simulink model "dwa_obstacle_avoidance"  (R2023b)
settings: Solver=VariableStepAuto  StartTime=0.0  StopTime=30  RelTol=1e-3
InitFcn:
  | if (isempty(target))
  | %load map
  | load exampleMaps simpleMap
  | mapMatrix = img_logical;
  | mapScale = 1;
  | 
  | % Max speed parameters
  | maxLinSpeed = 1.5;
  | maxAngle = deg2rad(45);
  | maxAngSpeed = 0.3;
  | 
  | % Initial pose of the robot
  | initX = 7;
  | initY = 22;
  | initTheta = pi;
  | v0=0;
  | w0=0;
  | 
  | % range sensor parameters
  | scanAngles = -pi/2:pi/128:pi/2;
  | maxRange = 12;
  | lidarNoiseVariance = 0.1^2;
  | lidarNoiseSeeds = randi(intmax,size(scanAngles));
  | 
  | %simulation parameters
  | sampleTime=0.05;
  | target = [25;5];
  | wheelBase=1.4;
  | end
values from neighbouring files (symbols this model uses):
  k1 = 0.80    (= 0.8)    [dynamic_window_init.m]    (also in sequence_dynamic_window_init.m = 0.9)
  k2 = 0.006    [dynamic_window_init.m]    (also in sequence_dynamic_window_init.m)
  k3 = 0.02    [dynamic_window_init.m]    (also in sequence_dynamic_window_init.m = 0.1)
libraries: robotmobilelib x1
settings Model: Creator=lucia  LastModifiedBy=lucia

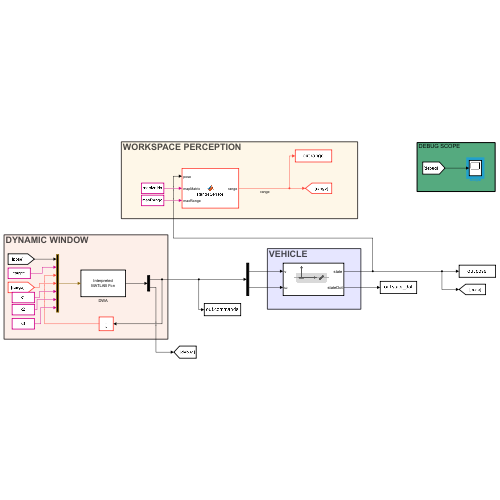
[thumbnail: Simulink's stored preview of the top-level diagram]
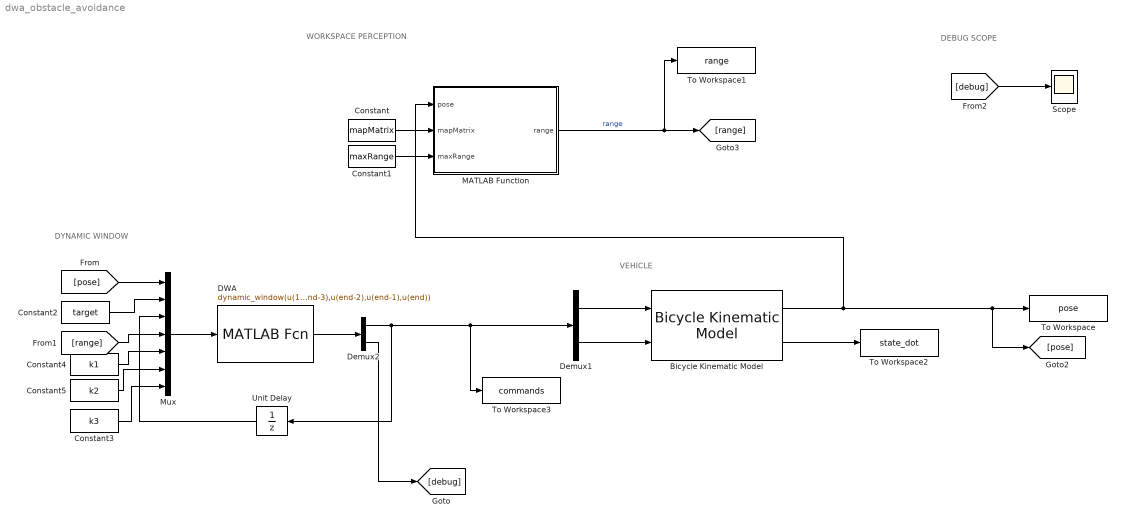
== system dwa_obstacle_avoidance ==
  note: DEBUG SCOPE
  note: DYNAMIC WINDOW
  note: VEHICLE
  note: WORKSPACE PERCEPTION
  Bicycle Kinematic Model : robotmobilelib/Bicycle Kinematic Model  VehicleInputs=Vehicle Speed & Heading Angular Velocity  WheelBase=wheelBase  VehicleSpeedRange=[0 maxLinSpeed]  MaxSteeringAngle=maxAngle  InitialState=[initX, initY, initTheta]  SimulateUsing=Interpreted execution
  Constant : Constant  Value=mapMatrix
  Constant1 : Constant  Value=maxRange
  Constant2 : Constant  Value=target
  Constant3 : Constant  Value=k3
  Constant4 : Constant  Value=k1
  Constant5 : Constant  Value=k2
  DWA : MATLABFcn  MATLABFcn=dynamic_window(u(1:3),u(4:5),u(6:7),u(8:end-3),u(end-2),u(end-1),u(end))  OutputDimensions=5
  Demux1 : Demux  Outputs=2
  Demux2 : Demux  Outputs=[2 3]
  MATLAB Function : MATLAB Function  TreatAsAtomicUnit=on
  Mux : Mux  Inputs=7
  Scope : Scope
  To Workspace : ToWorkspace  VariableName=pose  SampleTime=-1
      settings: Save2DSignal=2-D array (concatenate along first dimension)
  To Workspace1 : ToWorkspace  VariableName=range  SampleTime=-1
  To Workspace2 : ToWorkspace  VariableName=state_dot  SampleTime=-1
      settings: Save2DSignal=2-D array (concatenate along first dimension)
  To Workspace3 : ToWorkspace  VariableName=commands  SampleTime=-1
      settings: Save2DSignal=2-D array (concatenate along first dimension)
  Unit Delay : UnitDelay  InitialCondition=[v0; w0]  SampleTime=sampleTime  HasFrameUpgradeWarning=on
  wires:
  Bicycle Kinematic Model/1 -> MATLAB Function/1(pose), [pose], To Workspace/1
  Constant1/1 -> MATLAB Function/3(maxRange)
  Constant/1 -> MATLAB Function/2(mapMatrix)
  DWA/1 -> Demux2/1
  [pose] -> Mux/1
  [range] -> Mux/4
  Unit Delay/1 -> Mux/3
  Constant2/1 -> Mux/2
  Bicycle Kinematic Model/2 -> To Workspace2/1
  Demux2/1 -> Unit Delay/1, Demux1/1, To Workspace3/1
  Demux1/1 -> Bicycle Kinematic Model/1
  Mux/1 -> DWA/1
  MATLAB Function/1(range) -> To Workspace1/1, [range]  "range"
  Demux1/2 -> Bicycle Kinematic Model/2
  Demux2/2 -> [debug]
  [debug] -> Scope/1
  Constant4/1 -> Mux/5
  Constant5/1 -> Mux/6
  Constant3/1 -> Mux/7

== matlab function dwa_obstacle_avoidance/MATLAB Function ==
  settings: updateMethod=DISCRETE
  data: range output size=[129,1]; pose input size=[3, 1]; mapMatrix input size=[size(mapMatrix, 1), size(mapMatrix, 2)]; maxRange input; mapScale parameter
function range = RangeSensor(pose, mapMatrix, maxRange, mapScale)
% This function may be removed in the future.
% Copyright The MathWorks Inc, 2023
persistent r
 if isempty(r)
    r = rangeSensor('HorizontalAngle', [-pi/2,pi/2], 'HorizontalAngleResolution', pi/128, 'Range', [0 maxRange]);
end
map = binaryOccupancyMap(mapMatrix, 1);
p = pose';

% The range sensor accepts a pose on the map which is within the map's
% limits. Thus, filter out positions outside the map, and override them
% with readings that are zero.
xcord=p(:,1);
ycord=p(:,2);
xmin=map.XWorldLimits(1);
ymin=map.YWorldLimits(1);
xmax=map.XWorldLimits(2);
ymax=map.YWorldLimits(2);
isxvalid=xcord>=xmin&xcord<=xmax;
isyvalid=ycord>=ymin&ycord<=ymax;
isInside=isxvalid&isyvalid;
range = zeros(r.NumReadings,size(p,1));
range(:,isInside) = r(p(isInside,:), map);
%angles = -3*pi/8:pi/8:3*pi/8
end
